simulink library "P50_14s4pX10_rebuild"  (R2026a)
settings: Solver=VariableStepAuto
undefined symbols (not defined in the file or in its folder): battery_builder_rtmsupport, gcbh
libraries: nesl_utility x20, P50_14s4pX10_rebuild_lib x20
(part 2 of 2)

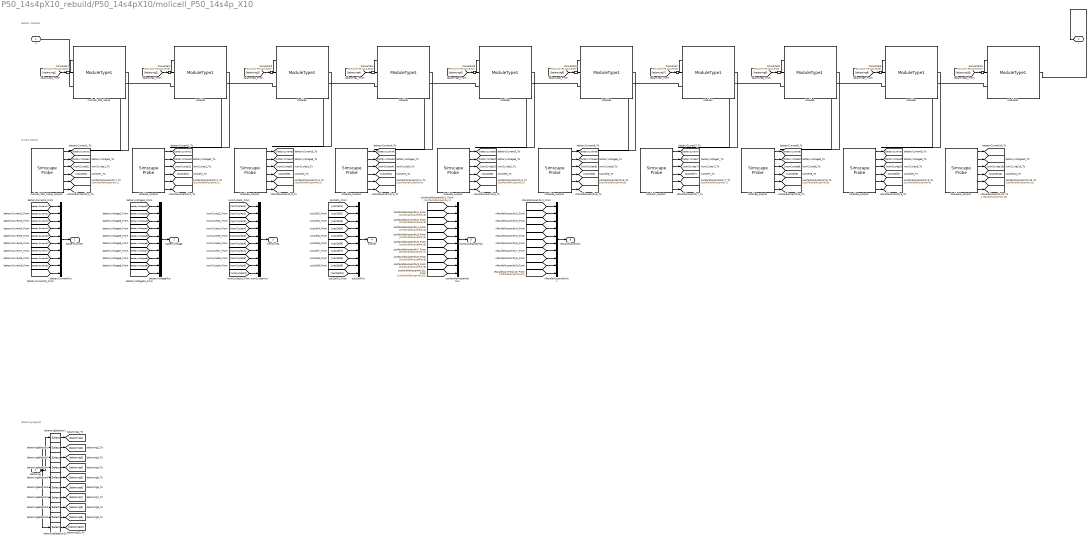
== system P50_14s4pX10_rebuild/P50_14s4pX10/molicell_P50_14s4p_X10 ==
  note: Balancing Signals
  note: Output Signals
  note: Battery Modules
  balancing : Inport  PortDimensions=140
  Converter{1..10} (10 alike) : nesl_utility/Simulink-PS Converter  PhysicalDomain=network_engine_domain  SubClassName=ps_input  LeftPortType=input  RightPortType=output  PseudoPeriodic=off  Frequencies=[]  NoiseDistribution=none  NoiseParameters=[]  Unit=1  AffineConversion=off  FilteringAndDerivatives=provide  SimscapeFilterOrder=1  InputFilterTimeConstant=0.001  UdotUserProvided=0
  Module10 : P50_14s4pX10_rebuild_lib/Modules/ModuleType1  BatteryCapacityCell=ModuleType1.BatteryCapacityCell A*hr  ExtrapolationMethodCell=simscape.enum.extrapolation.linear  SOCBreakpointsCell=ModuleType1.SOCBreakpointsCell  TemperatureBreakpointsCell=ModuleType1.TemperatureBreakpointsCell degC  OpenCircuitVoltageThermalCell=ModuleType1.OpenCircuitVoltageThermalCell V  VoltageRangeCell=ModuleType1.VoltageRangeCell V  ResistanceSOCBreakpointsCell=ModuleType1.ResistanceSOCBreakpointsCell  ResistanceTemperatureBreakpointsCell=ModuleType1.ResistanceTemperatureBreakpointsCell degC  R0ThermalCell=ModuleType1.R0ThermalCell Ohm  SimulationTemperatureCell=ModuleType1.SimulationTemperatureCell K  CellBalancingClosedResistance=ModuleType1.CellBalancingClosedResistance Ohm  CellBalancingOpenConductance=ModuleType1.CellBalancingOpenConductance 1/Ohm  CellBalancingThreshold=ModuleType1.CellBalancingThreshold  CellBalancingResistance=ModuleType1.CellBalancingResistance Ohm  socCell_specify=on  socCell_priority=High  socCell=molicell_P50_14s4p_X10.Module10.socCell  socCell_nominal_specify=off  socCell_nominal_value=1  socCell_nominal_unit=1  batteryVoltage_specify=on  batteryVoltage_priority=None  batteryVoltage=molicell_P50_14s4p_X10.Module10.batteryVoltage V  batteryVoltage_nominal_specify=off  batteryVoltage_nominal_value=1  batteryVoltage_nominal_unit=V  batteryCurrent_specify=on  batteryCurrent_priority=None  batteryCurrent=molicell_P50_14s4p_X10.Module10.batteryCurrent A  batteryCurrent_nominal_specify=off  batteryCurrent_nominal_value=1  batteryCurrent_nominal_unit=A  numCycles_specify=on  numCycles_priority=High  numCycles=molicell_P50_14s4p_X10.Module10.numCycles  numCycles_nominal_specify=off  numCycles_nominal_value=1  numCycles_nominal_unit=1  vParallelAssembly_specify=on  vParallelAssembly_priority=None  vParallelAssembly=molicell_P50_14s4p_X10.Module10.vParallelAssembly V  vParallelAssembly_nominal_specify=off  vParallelAssembly_nominal_value=1  vParallelAssembly_nominal_unit=V  socParallelAssembly_specify=on  socParallelAssembly_priority=None  socParallelAssembly=molicell_P50_14s4p_X10.Module10.socParallelAssembly  socParallelAssembly_nominal_specify=off  socParallelAssembly_nominal_value=1  socParallelAssembly_nominal_unit=1
  Module10_outputs : SimscapeProbe  BoundBlock=214  Variables="{\"batteryCurrent\":{\"Probing\":\"ON\"},\"batteryVoltage\":{\"Probing\":\"ON\"},\"numCycles\":{\"Probing\":\"ON\"},\"socCell\":{\"Probing\":\"ON\"},\"socParallelAssembly\":{\"Probing\":\"ON\"},\"vParallelAssembly\":{\"Probing\":\"ON\"}}"
  Module2 : P50_14s4pX10_rebuild_lib/Modules/ModuleType1  BatteryCapacityCell=ModuleType1.BatteryCapacityCell A*hr  ExtrapolationMethodCell=simscape.enum.extrapolation.linear  SOCBreakpointsCell=ModuleType1.SOCBreakpointsCell  TemperatureBreakpointsCell=ModuleType1.TemperatureBreakpointsCell degC  OpenCircuitVoltageThermalCell=ModuleType1.OpenCircuitVoltageThermalCell V  VoltageRangeCell=ModuleType1.VoltageRangeCell V  ResistanceSOCBreakpointsCell=ModuleType1.ResistanceSOCBreakpointsCell  ResistanceTemperatureBreakpointsCell=ModuleType1.ResistanceTemperatureBreakpointsCell degC  R0ThermalCell=ModuleType1.R0ThermalCell Ohm  SimulationTemperatureCell=ModuleType1.SimulationTemperatureCell K  CellBalancingClosedResistance=ModuleType1.CellBalancingClosedResistance Ohm  CellBalancingOpenConductance=ModuleType1.CellBalancingOpenConductance 1/Ohm  CellBalancingThreshold=ModuleType1.CellBalancingThreshold  CellBalancingResistance=ModuleType1.CellBalancingResistance Ohm  socCell_specify=on  socCell_priority=High  socCell=molicell_P50_14s4p_X10.Module2.socCell  socCell_nominal_specify=off  socCell_nominal_value=1  socCell_nominal_unit=1  batteryVoltage_specify=on  batteryVoltage_priority=None  batteryVoltage=molicell_P50_14s4p_X10.Module2.batteryVoltage V  batteryVoltage_nominal_specify=off  batteryVoltage_nominal_value=1  batteryVoltage_nominal_unit=V  batteryCurrent_specify=on  batteryCurrent_priority=None  batteryCurrent=molicell_P50_14s4p_X10.Module2.batteryCurrent A  batteryCurrent_nominal_specify=off  batteryCurrent_nominal_value=1  batteryCurrent_nominal_unit=A  numCycles_specify=on  numCycles_priority=High  numCycles=molicell_P50_14s4p_X10.Module2.numCycles  numCycles_nominal_specify=off  numCycles_nominal_value=1  numCycles_nominal_unit=1  vParallelAssembly_specify=on  vParallelAssembly_priority=None  vParallelAssembly=molicell_P50_14s4p_X10.Module2.vParallelAssembly V  vParallelAssembly_nominal_specify=off  vParallelAssembly_nominal_value=1  vParallelAssembly_nominal_unit=V  socParallelAssembly_specify=on  socParallelAssembly_priority=None  socParallelAssembly=molicell_P50_14s4p_X10.Module2.socParallelAssembly  socParallelAssembly_nominal_specify=off  socParallelAssembly_nominal_value=1  socParallelAssembly_nominal_unit=1
  Module2_outputs : SimscapeProbe  BoundBlock=216  Variables="{\"batteryCurrent\":{\"Probing\":\"ON\"},\"batteryVoltage\":{\"Probing\":\"ON\"},\"numCycles\":{\"Probing\":\"ON\"},\"socCell\":{\"Probing\":\"ON\"},\"socParallelAssembly\":{\"Probing\":\"ON\"},\"vParallelAssembly\":{\"Probing\":\"ON\"}}"
  Module3 : P50_14s4pX10_rebuild_lib/Modules/ModuleType1  BatteryCapacityCell=ModuleType1.BatteryCapacityCell A*hr  ExtrapolationMethodCell=simscape.enum.extrapolation.linear  SOCBreakpointsCell=ModuleType1.SOCBreakpointsCell  TemperatureBreakpointsCell=ModuleType1.TemperatureBreakpointsCell degC  OpenCircuitVoltageThermalCell=ModuleType1.OpenCircuitVoltageThermalCell V  VoltageRangeCell=ModuleType1.VoltageRangeCell V  ResistanceSOCBreakpointsCell=ModuleType1.ResistanceSOCBreakpointsCell  ResistanceTemperatureBreakpointsCell=ModuleType1.ResistanceTemperatureBreakpointsCell degC  R0ThermalCell=ModuleType1.R0ThermalCell Ohm  SimulationTemperatureCell=ModuleType1.SimulationTemperatureCell K  CellBalancingClosedResistance=ModuleType1.CellBalancingClosedResistance Ohm  CellBalancingOpenConductance=ModuleType1.CellBalancingOpenConductance 1/Ohm  CellBalancingThreshold=ModuleType1.CellBalancingThreshold  CellBalancingResistance=ModuleType1.CellBalancingResistance Ohm  socCell_specify=on  socCell_priority=High  socCell=molicell_P50_14s4p_X10.Module3.socCell  socCell_nominal_specify=off  socCell_nominal_value=1  socCell_nominal_unit=1  batteryVoltage_specify=on  batteryVoltage_priority=None  batteryVoltage=molicell_P50_14s4p_X10.Module3.batteryVoltage V  batteryVoltage_nominal_specify=off  batteryVoltage_nominal_value=1  batteryVoltage_nominal_unit=V  batteryCurrent_specify=on  batteryCurrent_priority=None  batteryCurrent=molicell_P50_14s4p_X10.Module3.batteryCurrent A  batteryCurrent_nominal_specify=off  batteryCurrent_nominal_value=1  batteryCurrent_nominal_unit=A  numCycles_specify=on  numCycles_priority=High  numCycles=molicell_P50_14s4p_X10.Module3.numCycles  numCycles_nominal_specify=off  numCycles_nominal_value=1  numCycles_nominal_unit=1  vParallelAssembly_specify=on  vParallelAssembly_priority=None  vParallelAssembly=molicell_P50_14s4p_X10.Module3.vParallelAssembly V  vParallelAssembly_nominal_specify=off  vParallelAssembly_nominal_value=1  vParallelAssembly_nominal_unit=V  socParallelAssembly_specify=on  socParallelAssembly_priority=None  socParallelAssembly=molicell_P50_14s4p_X10.Module3.socParallelAssembly  socParallelAssembly_nominal_specify=off  socParallelAssembly_nominal_value=1  socParallelAssembly_nominal_unit=1
  Module3_outputs : SimscapeProbe  BoundBlock=218  Variables="{\"batteryCurrent\":{\"Probing\":\"ON\"},\"batteryVoltage\":{\"Probing\":\"ON\"},\"numCycles\":{\"Probing\":\"ON\"},\"socCell\":{\"Probing\":\"ON\"},\"socParallelAssembly\":{\"Probing\":\"ON\"},\"vParallelAssembly\":{\"Probing\":\"ON\"}}"
  Module4 : P50_14s4pX10_rebuild_lib/Modules/ModuleType1  BatteryCapacityCell=ModuleType1.BatteryCapacityCell A*hr  ExtrapolationMethodCell=simscape.enum.extrapolation.linear  SOCBreakpointsCell=ModuleType1.SOCBreakpointsCell  TemperatureBreakpointsCell=ModuleType1.TemperatureBreakpointsCell degC  OpenCircuitVoltageThermalCell=ModuleType1.OpenCircuitVoltageThermalCell V  VoltageRangeCell=ModuleType1.VoltageRangeCell V  ResistanceSOCBreakpointsCell=ModuleType1.ResistanceSOCBreakpointsCell  ResistanceTemperatureBreakpointsCell=ModuleType1.ResistanceTemperatureBreakpointsCell degC  R0ThermalCell=ModuleType1.R0ThermalCell Ohm  SimulationTemperatureCell=ModuleType1.SimulationTemperatureCell K  CellBalancingClosedResistance=ModuleType1.CellBalancingClosedResistance Ohm  CellBalancingOpenConductance=ModuleType1.CellBalancingOpenConductance 1/Ohm  CellBalancingThreshold=ModuleType1.CellBalancingThreshold  CellBalancingResistance=ModuleType1.CellBalancingResistance Ohm  socCell_specify=on  socCell_priority=High  socCell=molicell_P50_14s4p_X10.Module4.socCell  socCell_nominal_specify=off  socCell_nominal_value=1  socCell_nominal_unit=1  batteryVoltage_specify=on  batteryVoltage_priority=None  batteryVoltage=molicell_P50_14s4p_X10.Module4.batteryVoltage V  batteryVoltage_nominal_specify=off  batteryVoltage_nominal_value=1  batteryVoltage_nominal_unit=V  batteryCurrent_specify=on  batteryCurrent_priority=None  batteryCurrent=molicell_P50_14s4p_X10.Module4.batteryCurrent A  batteryCurrent_nominal_specify=off  batteryCurrent_nominal_value=1  batteryCurrent_nominal_unit=A  numCycles_specify=on  numCycles_priority=High  numCycles=molicell_P50_14s4p_X10.Module4.numCycles  numCycles_nominal_specify=off  numCycles_nominal_value=1  numCycles_nominal_unit=1  vParallelAssembly_specify=on  vParallelAssembly_priority=None  vParallelAssembly=molicell_P50_14s4p_X10.Module4.vParallelAssembly V  vParallelAssembly_nominal_specify=off  vParallelAssembly_nominal_value=1  vParallelAssembly_nominal_unit=V  socParallelAssembly_specify=on  socParallelAssembly_priority=None  socParallelAssembly=molicell_P50_14s4p_X10.Module4.socParallelAssembly  socParallelAssembly_nominal_specify=off  socParallelAssembly_nominal_value=1  socParallelAssembly_nominal_unit=1
  Module4_outputs : SimscapeProbe  BoundBlock=220  Variables="{\"batteryCurrent\":{\"Probing\":\"ON\"},\"batteryVoltage\":{\"Probing\":\"ON\"},\"numCycles\":{\"Probing\":\"ON\"},\"socCell\":{\"Probing\":\"ON\"},\"socParallelAssembly\":{\"Probing\":\"ON\"},\"vParallelAssembly\":{\"Probing\":\"ON\"}}"
  Module5 : P50_14s4pX10_rebuild_lib/Modules/ModuleType1  BatteryCapacityCell=ModuleType1.BatteryCapacityCell A*hr  ExtrapolationMethodCell=simscape.enum.extrapolation.linear  SOCBreakpointsCell=ModuleType1.SOCBreakpointsCell  TemperatureBreakpointsCell=ModuleType1.TemperatureBreakpointsCell degC  OpenCircuitVoltageThermalCell=ModuleType1.OpenCircuitVoltageThermalCell V  VoltageRangeCell=ModuleType1.VoltageRangeCell V  ResistanceSOCBreakpointsCell=ModuleType1.ResistanceSOCBreakpointsCell  ResistanceTemperatureBreakpointsCell=ModuleType1.ResistanceTemperatureBreakpointsCell degC  R0ThermalCell=ModuleType1.R0ThermalCell Ohm  SimulationTemperatureCell=ModuleType1.SimulationTemperatureCell K  CellBalancingClosedResistance=ModuleType1.CellBalancingClosedResistance Ohm  CellBalancingOpenConductance=ModuleType1.CellBalancingOpenConductance 1/Ohm  CellBalancingThreshold=ModuleType1.CellBalancingThreshold  CellBalancingResistance=ModuleType1.CellBalancingResistance Ohm  socCell_specify=on  socCell_priority=High  socCell=molicell_P50_14s4p_X10.Module5.socCell  socCell_nominal_specify=off  socCell_nominal_value=1  socCell_nominal_unit=1  batteryVoltage_specify=on  batteryVoltage_priority=None  batteryVoltage=molicell_P50_14s4p_X10.Module5.batteryVoltage V  batteryVoltage_nominal_specify=off  batteryVoltage_nominal_value=1  batteryVoltage_nominal_unit=V  batteryCurrent_specify=on  batteryCurrent_priority=None  batteryCurrent=molicell_P50_14s4p_X10.Module5.batteryCurrent A  batteryCurrent_nominal_specify=off  batteryCurrent_nominal_value=1  batteryCurrent_nominal_unit=A  numCycles_specify=on  numCycles_priority=High  numCycles=molicell_P50_14s4p_X10.Module5.numCycles  numCycles_nominal_specify=off  numCycles_nominal_value=1  numCycles_nominal_unit=1  vParallelAssembly_specify=on  vParallelAssembly_priority=None  vParallelAssembly=molicell_P50_14s4p_X10.Module5.vParallelAssembly V  vParallelAssembly_nominal_specify=off  vParallelAssembly_nominal_value=1  vParallelAssembly_nominal_unit=V  socParallelAssembly_specify=on  socParallelAssembly_priority=None  socParallelAssembly=molicell_P50_14s4p_X10.Module5.socParallelAssembly  socParallelAssembly_nominal_specify=off  socParallelAssembly_nominal_value=1  socParallelAssembly_nominal_unit=1
  Module5_outputs : SimscapeProbe  BoundBlock=222  Variables="{\"batteryCurrent\":{\"Probing\":\"ON\"},\"batteryVoltage\":{\"Probing\":\"ON\"},\"numCycles\":{\"Probing\":\"ON\"},\"socCell\":{\"Probing\":\"ON\"},\"socParallelAssembly\":{\"Probing\":\"ON\"},\"vParallelAssembly\":{\"Probing\":\"ON\"}}"
  Module6 : P50_14s4pX10_rebuild_lib/Modules/ModuleType1  BatteryCapacityCell=ModuleType1.BatteryCapacityCell A*hr  ExtrapolationMethodCell=simscape.enum.extrapolation.linear  SOCBreakpointsCell=ModuleType1.SOCBreakpointsCell  TemperatureBreakpointsCell=ModuleType1.TemperatureBreakpointsCell degC  OpenCircuitVoltageThermalCell=ModuleType1.OpenCircuitVoltageThermalCell V  VoltageRangeCell=ModuleType1.VoltageRangeCell V  ResistanceSOCBreakpointsCell=ModuleType1.ResistanceSOCBreakpointsCell  ResistanceTemperatureBreakpointsCell=ModuleType1.ResistanceTemperatureBreakpointsCell degC  R0ThermalCell=ModuleType1.R0ThermalCell Ohm  SimulationTemperatureCell=ModuleType1.SimulationTemperatureCell K  CellBalancingClosedResistance=ModuleType1.CellBalancingClosedResistance Ohm  CellBalancingOpenConductance=ModuleType1.CellBalancingOpenConductance 1/Ohm  CellBalancingThreshold=ModuleType1.CellBalancingThreshold  CellBalancingResistance=ModuleType1.CellBalancingResistance Ohm  socCell_specify=on  socCell_priority=High  socCell=molicell_P50_14s4p_X10.Module6.socCell  socCell_nominal_specify=off  socCell_nominal_value=1  socCell_nominal_unit=1  batteryVoltage_specify=on  batteryVoltage_priority=None  batteryVoltage=molicell_P50_14s4p_X10.Module6.batteryVoltage V  batteryVoltage_nominal_specify=off  batteryVoltage_nominal_value=1  batteryVoltage_nominal_unit=V  batteryCurrent_specify=on  batteryCurrent_priority=None  batteryCurrent=molicell_P50_14s4p_X10.Module6.batteryCurrent A  batteryCurrent_nominal_specify=off  batteryCurrent_nominal_value=1  batteryCurrent_nominal_unit=A  numCycles_specify=on  numCycles_priority=High  numCycles=molicell_P50_14s4p_X10.Module6.numCycles  numCycles_nominal_specify=off  numCycles_nominal_value=1  numCycles_nominal_unit=1  vParallelAssembly_specify=on  vParallelAssembly_priority=None  vParallelAssembly=molicell_P50_14s4p_X10.Module6.vParallelAssembly V  vParallelAssembly_nominal_specify=off  vParallelAssembly_nominal_value=1  vParallelAssembly_nominal_unit=V  socParallelAssembly_specify=on  socParallelAssembly_priority=None  socParallelAssembly=molicell_P50_14s4p_X10.Module6.socParallelAssembly  socParallelAssembly_nominal_specify=off  socParallelAssembly_nominal_value=1  socParallelAssembly_nominal_unit=1
  Module6_outputs : SimscapeProbe  BoundBlock=224  Variables="{\"batteryCurrent\":{\"Probing\":\"ON\"},\"batteryVoltage\":{\"Probing\":\"ON\"},\"numCycles\":{\"Probing\":\"ON\"},\"socCell\":{\"Probing\":\"ON\"},\"socParallelAssembly\":{\"Probing\":\"ON\"},\"vParallelAssembly\":{\"Probing\":\"ON\"}}"
  Module7 : P50_14s4pX10_rebuild_lib/Modules/ModuleType1  BatteryCapacityCell=ModuleType1.BatteryCapacityCell A*hr  ExtrapolationMethodCell=simscape.enum.extrapolation.linear  SOCBreakpointsCell=ModuleType1.SOCBreakpointsCell  TemperatureBreakpointsCell=ModuleType1.TemperatureBreakpointsCell degC  OpenCircuitVoltageThermalCell=ModuleType1.OpenCircuitVoltageThermalCell V  VoltageRangeCell=ModuleType1.VoltageRangeCell V  ResistanceSOCBreakpointsCell=ModuleType1.ResistanceSOCBreakpointsCell  ResistanceTemperatureBreakpointsCell=ModuleType1.ResistanceTemperatureBreakpointsCell degC  R0ThermalCell=ModuleType1.R0ThermalCell Ohm  SimulationTemperatureCell=ModuleType1.SimulationTemperatureCell K  CellBalancingClosedResistance=ModuleType1.CellBalancingClosedResistance Ohm  CellBalancingOpenConductance=ModuleType1.CellBalancingOpenConductance 1/Ohm  CellBalancingThreshold=ModuleType1.CellBalancingThreshold  CellBalancingResistance=ModuleType1.CellBalancingResistance Ohm  socCell_specify=on  socCell_priority=High  socCell=molicell_P50_14s4p_X10.Module7.socCell  socCell_nominal_specify=off  socCell_nominal_value=1  socCell_nominal_unit=1  batteryVoltage_specify=on  batteryVoltage_priority=None  batteryVoltage=molicell_P50_14s4p_X10.Module7.batteryVoltage V  batteryVoltage_nominal_specify=off  batteryVoltage_nominal_value=1  batteryVoltage_nominal_unit=V  batteryCurrent_specify=on  batteryCurrent_priority=None  batteryCurrent=molicell_P50_14s4p_X10.Module7.batteryCurrent A  batteryCurrent_nominal_specify=off  batteryCurrent_nominal_value=1  batteryCurrent_nominal_unit=A  numCycles_specify=on  numCycles_priority=High  numCycles=molicell_P50_14s4p_X10.Module7.numCycles  numCycles_nominal_specify=off  numCycles_nominal_value=1  numCycles_nominal_unit=1  vParallelAssembly_specify=on  vParallelAssembly_priority=None  vParallelAssembly=molicell_P50_14s4p_X10.Module7.vParallelAssembly V  vParallelAssembly_nominal_specify=off  vParallelAssembly_nominal_value=1  vParallelAssembly_nominal_unit=V  socParallelAssembly_specify=on  socParallelAssembly_priority=None  socParallelAssembly=molicell_P50_14s4p_X10.Module7.socParallelAssembly  socParallelAssembly_nominal_specify=off  socParallelAssembly_nominal_value=1  socParallelAssembly_nominal_unit=1
  Module7_outputs : SimscapeProbe  BoundBlock=226  Variables="{\"batteryCurrent\":{\"Probing\":\"ON\"},\"batteryVoltage\":{\"Probing\":\"ON\"},\"numCycles\":{\"Probing\":\"ON\"},\"socCell\":{\"Probing\":\"ON\"},\"socParallelAssembly\":{\"Probing\":\"ON\"},\"vParallelAssembly\":{\"Probing\":\"ON\"}}"
  Module8 : P50_14s4pX10_rebuild_lib/Modules/ModuleType1  BatteryCapacityCell=ModuleType1.BatteryCapacityCell A*hr  ExtrapolationMethodCell=simscape.enum.extrapolation.linear  SOCBreakpointsCell=ModuleType1.SOCBreakpointsCell  TemperatureBreakpointsCell=ModuleType1.TemperatureBreakpointsCell degC  OpenCircuitVoltageThermalCell=ModuleType1.OpenCircuitVoltageThermalCell V  VoltageRangeCell=ModuleType1.VoltageRangeCell V  ResistanceSOCBreakpointsCell=ModuleType1.ResistanceSOCBreakpointsCell  ResistanceTemperatureBreakpointsCell=ModuleType1.ResistanceTemperatureBreakpointsCell degC  R0ThermalCell=ModuleType1.R0ThermalCell Ohm  SimulationTemperatureCell=ModuleType1.SimulationTemperatureCell K  CellBalancingClosedResistance=ModuleType1.CellBalancingClosedResistance Ohm  CellBalancingOpenConductance=ModuleType1.CellBalancingOpenConductance 1/Ohm  CellBalancingThreshold=ModuleType1.CellBalancingThreshold  CellBalancingResistance=ModuleType1.CellBalancingResistance Ohm  socCell_specify=on  socCell_priority=High  socCell=molicell_P50_14s4p_X10.Module8.socCell  socCell_nominal_specify=off  socCell_nominal_value=1  socCell_nominal_unit=1  batteryVoltage_specify=on  batteryVoltage_priority=None  batteryVoltage=molicell_P50_14s4p_X10.Module8.batteryVoltage V  batteryVoltage_nominal_specify=off  batteryVoltage_nominal_value=1  batteryVoltage_nominal_unit=V  batteryCurrent_specify=on  batteryCurrent_priority=None  batteryCurrent=molicell_P50_14s4p_X10.Module8.batteryCurrent A  batteryCurrent_nominal_specify=off  batteryCurrent_nominal_value=1  batteryCurrent_nominal_unit=A  numCycles_specify=on  numCycles_priority=High  numCycles=molicell_P50_14s4p_X10.Module8.numCycles  numCycles_nominal_specify=off  numCycles_nominal_value=1  numCycles_nominal_unit=1  vParallelAssembly_specify=on  vParallelAssembly_priority=None  vParallelAssembly=molicell_P50_14s4p_X10.Module8.vParallelAssembly V  vParallelAssembly_nominal_specify=off  vParallelAssembly_nominal_value=1  vParallelAssembly_nominal_unit=V  socParallelAssembly_specify=on  socParallelAssembly_priority=None  socParallelAssembly=molicell_P50_14s4p_X10.Module8.socParallelAssembly  socParallelAssembly_nominal_specify=off  socParallelAssembly_nominal_value=1  socParallelAssembly_nominal_unit=1
  Module8_outputs : SimscapeProbe  BoundBlock=228  Variables="{\"batteryCurrent\":{\"Probing\":\"ON\"},\"batteryVoltage\":{\"Probing\":\"ON\"},\"numCycles\":{\"Probing\":\"ON\"},\"socCell\":{\"Probing\":\"ON\"},\"socParallelAssembly\":{\"Probing\":\"ON\"},\"vParallelAssembly\":{\"Probing\":\"ON\"}}"
  Module9 : P50_14s4pX10_rebuild_lib/Modules/ModuleType1  BatteryCapacityCell=ModuleType1.BatteryCapacityCell A*hr  ExtrapolationMethodCell=simscape.enum.extrapolation.linear  SOCBreakpointsCell=ModuleType1.SOCBreakpointsCell  TemperatureBreakpointsCell=ModuleType1.TemperatureBreakpointsCell degC  OpenCircuitVoltageThermalCell=ModuleType1.OpenCircuitVoltageThermalCell V  VoltageRangeCell=ModuleType1.VoltageRangeCell V  ResistanceSOCBreakpointsCell=ModuleType1.ResistanceSOCBreakpointsCell  ResistanceTemperatureBreakpointsCell=ModuleType1.ResistanceTemperatureBreakpointsCell degC  R0ThermalCell=ModuleType1.R0ThermalCell Ohm  SimulationTemperatureCell=ModuleType1.SimulationTemperatureCell K  CellBalancingClosedResistance=ModuleType1.CellBalancingClosedResistance Ohm  CellBalancingOpenConductance=ModuleType1.CellBalancingOpenConductance 1/Ohm  CellBalancingThreshold=ModuleType1.CellBalancingThreshold  CellBalancingResistance=ModuleType1.CellBalancingResistance Ohm  socCell_specify=on  socCell_priority=High  socCell=molicell_P50_14s4p_X10.Module9.socCell  socCell_nominal_specify=off  socCell_nominal_value=1  socCell_nominal_unit=1  batteryVoltage_specify=on  batteryVoltage_priority=None  batteryVoltage=molicell_P50_14s4p_X10.Module9.batteryVoltage V  batteryVoltage_nominal_specify=off  batteryVoltage_nominal_value=1  batteryVoltage_nominal_unit=V  batteryCurrent_specify=on  batteryCurrent_priority=None  batteryCurrent=molicell_P50_14s4p_X10.Module9.batteryCurrent A  batteryCurrent_nominal_specify=off  batteryCurrent_nominal_value=1  batteryCurrent_nominal_unit=A  numCycles_specify=on  numCycles_priority=High  numCycles=molicell_P50_14s4p_X10.Module9.numCycles  numCycles_nominal_specify=off  numCycles_nominal_value=1  numCycles_nominal_unit=1  vParallelAssembly_specify=on  vParallelAssembly_priority=None  vParallelAssembly=molicell_P50_14s4p_X10.Module9.vParallelAssembly V  vParallelAssembly_nominal_specify=off  vParallelAssembly_nominal_value=1  vParallelAssembly_nominal_unit=V  socParallelAssembly_specify=on  socParallelAssembly_priority=None  socParallelAssembly=molicell_P50_14s4p_X10.Module9.socParallelAssembly  socParallelAssembly_nominal_specify=off  socParallelAssembly_nominal_value=1  socParallelAssembly_nominal_unit=1
  Module9_outputs : SimscapeProbe  BoundBlock=230  Variables="{\"batteryCurrent\":{\"Probing\":\"ON\"},\"batteryVoltage\":{\"Probing\":\"ON\"},\"numCycles\":{\"Probing\":\"ON\"},\"socCell\":{\"Probing\":\"ON\"},\"socParallelAssembly\":{\"Probing\":\"ON\"},\"vParallelAssembly\":{\"Probing\":\"ON\"}}"
  balancingSelector1 : Selector  InputPortWidth=140  IndexOptions=Index vector (dialog)  Indices="[1   2   3   4   5   6   7   8   9  10  11  12  13  14]"  OutputSizes=1
  balancingSelector10 : Selector  InputPortWidth=140  IndexOptions=Index vector (dialog)  Indices="[127  128  129  130  131  132  133  134  135  136  137  138  139  140]"  OutputSizes=1
  balancingSelector2 : Selector  InputPortWidth=140  IndexOptions=Index vector (dialog)  Indices="[15  16  17  18  19  20  21  22  23  24  25  26  27  28]"  OutputSizes=1
  balancingSelector3 : Selector  InputPortWidth=140  IndexOptions=Index vector (dialog)  Indices="[29  30  31  32  33  34  35  36  37  38  39  40  41  42]"  OutputSizes=1
  balancingSelector4 : Selector  InputPortWidth=140  IndexOptions=Index vector (dialog)  Indices="[43  44  45  46  47  48  49  50  51  52  53  54  55  56]"  OutputSizes=1
  balancingSelector5 : Selector  InputPortWidth=140  IndexOptions=Index vector (dialog)  Indices="[57  58  59  60  61  62  63  64  65  66  67  68  69  70]"  OutputSizes=1
  balancingSelector6 : Selector  InputPortWidth=140  IndexOptions=Index vector (dialog)  Indices="[71  72  73  74  75  76  77  78  79  80  81  82  83  84]"  OutputSizes=1
  balancingSelector7 : Selector  InputPortWidth=140  IndexOptions=Index vector (dialog)  Indices="[85  86  87  88  89  90  91  92  93  94  95  96  97  98]"  OutputSizes=1
  balancingSelector8 : Selector  InputPortWidth=140  IndexOptions=Index vector (dialog)  Indices="[99  100  101  102  103  104  105  106  107  108  109  110  111  112]"  OutputSizes=1
  balancingSelector9 : Selector  InputPortWidth=140  IndexOptions=Index vector (dialog)  Indices="[113  114  115  116  117  118  119  120  121  122  123  124  125  126]"  OutputSizes=1
  batteryCurrentMux : Mux  Inputs=10
  batteryVoltageMux : Mux  Inputs=10
  molicell_P50_14s4p : P50_14s4pX10_rebuild_lib/Modules/ModuleType1  BatteryCapacityCell=ModuleType1.BatteryCapacityCell A*hr  ExtrapolationMethodCell=simscape.enum.extrapolation.linear  SOCBreakpointsCell=ModuleType1.SOCBreakpointsCell  TemperatureBreakpointsCell=ModuleType1.TemperatureBreakpointsCell degC  OpenCircuitVoltageThermalCell=ModuleType1.OpenCircuitVoltageThermalCell V  VoltageRangeCell=ModuleType1.VoltageRangeCell V  ResistanceSOCBreakpointsCell=ModuleType1.ResistanceSOCBreakpointsCell  ResistanceTemperatureBreakpointsCell=ModuleType1.ResistanceTemperatureBreakpointsCell degC  R0ThermalCell=ModuleType1.R0ThermalCell Ohm  SimulationTemperatureCell=ModuleType1.SimulationTemperatureCell K  CellBalancingClosedResistance=ModuleType1.CellBalancingClosedResistance Ohm  CellBalancingOpenConductance=ModuleType1.CellBalancingOpenConductance 1/Ohm  CellBalancingThreshold=ModuleType1.CellBalancingThreshold  CellBalancingResistance=ModuleType1.CellBalancingResistance Ohm  socCell_specify=on  socCell_priority=High  socCell=molicell_P50_14s4p_X10.molicell_P50_14s4p.socCell  socCell_nominal_specify=off  socCell_nominal_value=1  socCell_nominal_unit=1  batteryVoltage_specify=on  batteryVoltage_priority=None  batteryVoltage=molicell_P50_14s4p_X10.molicell_P50_14s4p.batteryVoltage V  batteryVoltage_nominal_specify=off  batteryVoltage_nominal_value=1  batteryVoltage_nominal_unit=V  batteryCurrent_specify=on  batteryCurrent_priority=None  batteryCurrent=molicell_P50_14s4p_X10.molicell_P50_14s4p.batteryCurrent A  batteryCurrent_nominal_specify=off  batteryCurrent_nominal_value=1  batteryCurrent_nominal_unit=A  numCycles_specify=on  numCycles_priority=High  numCycles=molicell_P50_14s4p_X10.molicell_P50_14s4p.numCycles  numCycles_nominal_specify=off  numCycles_nominal_value=1  numCycles_nominal_unit=1  vParallelAssembly_specify=on  vParallelAssembly_priority=None  vParallelAssembly=molicell_P50_14s4p_X10.molicell_P50_14s4p.vParallelAssembly V  vParallelAssembly_nominal_specify=off  vParallelAssembly_nominal_value=1  vParallelAssembly_nominal_unit=V  socParallelAssembly_specify=on  socParallelAssembly_priority=None  socParallelAssembly=molicell_P50_14s4p_X10.molicell_P50_14s4p.socParallelAssembly  socParallelAssembly_nominal_specify=off  socParallelAssembly_nominal_value=1  socParallelAssembly_nominal_unit=1
  molicell_P50_14s4p_outputs : SimscapeProbe  BoundBlock=304  Variables="{\"batteryCurrent\":{\"Probing\":\"ON\"},\"batteryVoltage\":{\"Probing\":\"ON\"},\"numCycles\":{\"Probing\":\"ON\"},\"socCell\":{\"Probing\":\"ON\"},\"socParallelAssembly\":{\"Probing\":\"ON\"},\"vParallelAssembly\":{\"Probing\":\"ON\"}}"
  numCyclesMux : Mux  Inputs=10
  socCellMux : Mux  Inputs=10
  socParallelAssemblyMux : Mux  Inputs=10
  vParallelAssemblyMux : Mux  Inputs=10
  + : PMIOPort  Side=Left
  - : PMIOPort  Port=2  Side=Right
  batteryCurrent : Outport
  batteryVoltage : Outport  Port=2
  numCycles : Outport  Port=3
  socCell : Outport  Port=4
  socParallelAssembly : Outport  Port=5
  vParallelAssembly : Outport  Port=6
  wires:
  balancingSelector10/1 -> [balancing10]
  [balancing10] -> Converter10/1
  balancingSelector9/1 -> [balancing9]
  [balancing9] -> Converter9/1
  balancingSelector8/1 -> [balancing8]
  [balancing8] -> Converter8/1
  balancingSelector7/1 -> [balancing7]
  [balancing7] -> Converter7/1
  balancingSelector6/1 -> [balancing6]
  [balancing6] -> Converter6/1
  balancingSelector5/1 -> [balancing5]
  [balancing5] -> Converter5/1
  balancingSelector4/1 -> [balancing4]
  [balancing4] -> Converter4/1
  balancingSelector3/1 -> [balancing3]
  [balancing3] -> Converter3/1
  balancingSelector2/1 -> [balancing2]
  [balancing2] -> Converter2/1
  balancingSelector1/1 -> [balancing1]
  balancing/1 -> balancingSelector10/1, balancingSelector9/1, balancingSelector8/1, balancingSelector7/1, balancingSelector6/1, balancingSelector5/1, balancingSelector4/1, balancingSelector3/1, balancingSelector2/1, balancingSelector1/1
  [balancing1] -> Converter1/1
  [vParallelAssembly10] -> vParallelAssemblyMux/10
  Module10_outputs/6 -> [vParallelAssembly10]
  [socParallelAssembly10] -> socParallelAssemblyMux/10
  Module10_outputs/5 -> [socParallelAssembly10]
  [socCell10] -> socCellMux/10
  Module10_outputs/4 -> [socCell10]
  [numCycles10] -> numCyclesMux/10
  Module10_outputs/3 -> [numCycles10]
  [batteryVoltage10] -> batteryVoltageMux/10
  Module10_outputs/2 -> [batteryVoltage10]
  [batteryCurrent10] -> batteryCurrentMux/10
  Module10_outputs/1 -> [batteryCurrent10]
  [vParallelAssembly9] -> vParallelAssemblyMux/9
  Module9_outputs/6 -> [vParallelAssembly9]
  [socParallelAssembly9] -> socParallelAssemblyMux/9
  Module9_outputs/5 -> [socParallelAssembly9]
  [socCell9] -> socCellMux/9
  Module9_outputs/4 -> [socCell9]
  [numCycles9] -> numCyclesMux/9
  Module9_outputs/3 -> [numCycles9]
  [batteryVoltage9] -> batteryVoltageMux/9
  Module9_outputs/2 -> [batteryVoltage9]
  [batteryCurrent9] -> batteryCurrentMux/9
  Module9_outputs/1 -> [batteryCurrent9]
  [vParallelAssembly8] -> vParallelAssemblyMux/8
  Module8_outputs/6 -> [vParallelAssembly8]
  [socParallelAssembly8] -> socParallelAssemblyMux/8
  Module8_outputs/5 -> [socParallelAssembly8]
  [socCell8] -> socCellMux/8
  Module8_outputs/4 -> [socCell8]
  [numCycles8] -> numCyclesMux/8
  Module8_outputs/3 -> [numCycles8]
  [batteryVoltage8] -> batteryVoltageMux/8
  Module8_outputs/2 -> [batteryVoltage8]
  [batteryCurrent8] -> batteryCurrentMux/8
  Module8_outputs/1 -> [batteryCurrent8]
  [vParallelAssembly7] -> vParallelAssemblyMux/7
  Module7_outputs/6 -> [vParallelAssembly7]
  [socParallelAssembly7] -> socParallelAssemblyMux/7
  Module7_outputs/5 -> [socParallelAssembly7]
  [socCell7] -> socCellMux/7
  Module7_outputs/4 -> [socCell7]
  [numCycles7] -> numCyclesMux/7
  Module7_outputs/3 -> [numCycles7]
  [batteryVoltage7] -> batteryVoltageMux/7
  Module7_outputs/2 -> [batteryVoltage7]
  [batteryCurrent7] -> batteryCurrentMux/7
  Module7_outputs/1 -> [batteryCurrent7]
  [vParallelAssembly6] -> vParallelAssemblyMux/6
  Module6_outputs/6 -> [vParallelAssembly6]
  [socParallelAssembly6] -> socParallelAssemblyMux/6
  Module6_outputs/5 -> [socParallelAssembly6]
  [socCell6] -> socCellMux/6
  Module6_outputs/4 -> [socCell6]
  [numCycles6] -> numCyclesMux/6
  Module6_outputs/3 -> [numCycles6]
  [batteryVoltage6] -> batteryVoltageMux/6
  Module6_outputs/2 -> [batteryVoltage6]
  [batteryCurrent6] -> batteryCurrentMux/6
  Module6_outputs/1 -> [batteryCurrent6]
  [vParallelAssembly5] -> vParallelAssemblyMux/5
  Module5_outputs/6 -> [vParallelAssembly5]
  [socParallelAssembly5] -> socParallelAssemblyMux/5
  Module5_outputs/5 -> [socParallelAssembly5]
  [socCell5] -> socCellMux/5
  Module5_outputs/4 -> [socCell5]
  [numCycles5] -> numCyclesMux/5
  Module5_outputs/3 -> [numCycles5]
  [batteryVoltage5] -> batteryVoltageMux/5
  Module5_outputs/2 -> [batteryVoltage5]
  [batteryCurrent5] -> batteryCurrentMux/5
  Module5_outputs/1 -> [batteryCurrent5]
  [vParallelAssembly4] -> vParallelAssemblyMux/4
  Module4_outputs/6 -> [vParallelAssembly4]
  [socParallelAssembly4] -> socParallelAssemblyMux/4
  Module4_outputs/5 -> [socParallelAssembly4]
  [socCell4] -> socCellMux/4
  Module4_outputs/4 -> [socCell4]
  [numCycles4] -> numCyclesMux/4
  Module4_outputs/3 -> [numCycles4]
  [batteryVoltage4] -> batteryVoltageMux/4
  Module4_outputs/2 -> [batteryVoltage4]
  [batteryCurrent4] -> batteryCurrentMux/4
  Module4_outputs/1 -> [batteryCurrent4]
  [vParallelAssembly3] -> vParallelAssemblyMux/3
  Module3_outputs/6 -> [vParallelAssembly3]
  [socParallelAssembly3] -> socParallelAssemblyMux/3
  Module3_outputs/5 -> [socParallelAssembly3]
  [socCell3] -> socCellMux/3
  Module3_outputs/4 -> [socCell3]
  [numCycles3] -> numCyclesMux/3
  Module3_outputs/3 -> [numCycles3]
  [batteryVoltage3] -> batteryVoltageMux/3
  Module3_outputs/2 -> [batteryVoltage3]
  [batteryCurrent3] -> batteryCurrentMux/3
  Module3_outputs/1 -> [batteryCurrent3]
  [vParallelAssembly2] -> vParallelAssemblyMux/2
  Module2_outputs/6 -> [vParallelAssembly2]
  [socParallelAssembly2] -> socParallelAssemblyMux/2
  Module2_outputs/5 -> [socParallelAssembly2]
  [socCell2] -> socCellMux/2
  Module2_outputs/4 -> [socCell2]
  [numCycles2] -> numCyclesMux/2
  Module2_outputs/3 -> [numCycles2]
  [batteryVoltage2] -> batteryVoltageMux/2
  Module2_outputs/2 -> [batteryVoltage2]
  [batteryCurrent2] -> batteryCurrentMux/2
  Module2_outputs/1 -> [batteryCurrent2]
  [vParallelAssembly1] -> vParallelAssemblyMux/1
  vParallelAssemblyMux/1 -> vParallelAssembly/1
  molicell_P50_14s4p_outputs/6 -> [vParallelAssembly1]
  [socParallelAssembly1] -> socParallelAssemblyMux/1
  socParallelAssemblyMux/1 -> socParallelAssembly/1
  molicell_P50_14s4p_outputs/5 -> [socParallelAssembly1]
  [socCell1] -> socCellMux/1
  socCellMux/1 -> socCell/1
  molicell_P50_14s4p_outputs/4 -> [socCell1]
  [numCycles1] -> numCyclesMux/1
  numCyclesMux/1 -> numCycles/1
  molicell_P50_14s4p_outputs/3 -> [numCycles1]
  [batteryVoltage1] -> batteryVoltageMux/1
  batteryVoltageMux/1 -> batteryVoltage/1
  molicell_P50_14s4p_outputs/2 -> [batteryVoltage1]
  [batteryCurrent1] -> batteryCurrentMux/1
  batteryCurrentMux/1 -> batteryCurrent/1
  molicell_P50_14s4p_outputs/1 -> [batteryCurrent1]
  connections:
  Converter10/RConn1 -- Module10/LConn1
  Converter9/RConn1 -- Module9/LConn1
  Converter8/RConn1 -- Module8/LConn1
  Converter7/RConn1 -- Module7/LConn1
  Converter6/RConn1 -- Module6/LConn1
  Converter5/RConn1 -- Module5/LConn1
  Converter4/RConn1 -- Module4/LConn1
  Converter3/RConn1 -- Module3/LConn1
  Converter2/RConn1 -- Module2/LConn1
  Converter1/RConn1 -- molicell_P50_14s4p/LConn1
  Module10/RConn1 -- -/RConn1
  molicell_P50_14s4p/LConn2 -- +/RConn1
  Module10/LConn2 -- Module9/RConn1
  Module9/LConn2 -- Module8/RConn1
  Module8/LConn2 -- Module7/RConn1
  Module7/LConn2 -- Module6/RConn1
  Module6/LConn2 -- Module5/RConn1
  Module5/LConn2 -- Module4/RConn1
  Module4/LConn2 -- Module3/RConn1
  Module3/LConn2 -- Module2/RConn1
  Module2/LConn2 -- molicell_P50_14s4p/RConn1
